simulink model "HeatExchanger_digital"  (Simulink 8.1)
settings: Solver=ode4  StartTime=0.0  StopTime=250  FixedStep=delta_t  RelTol=1e-3
values from neighbouring files (symbols this model uses):
  delta_t = 1 / sensor_sampling_rate    (= 0.1)    [HeatExchanger_ps.m]
  ki = 1.2    [HeatExchanger_ps.m]    (also in hxpumpcode.m = 1; hxpumpcodesanity.m; noErrornoDelay.mat = 1)
  kp = 4.995    [HeatExchanger_ps.m]    (also in hxpumpcode.m = 4; hxpumpcodesanity.m; noErrornoDelay.mat = 4)
  Sv_mh = 0.05    [HeatExchanger_ps.m]    (also in hxpumpcode.m = params.Sv_mh; hxpumpcodesanity.m; noErrornoDelay.mat)
  Sv_thi = 5e-2    (= 0.05)    [HeatExchanger_ps.m]    (also in hxpumpcode.m = params.Sv_thi; hxpumpcodesanity.m; noErrornoDelay.mat)
  Sv_tho = 0.1    [HeatExchanger_ps.m]    (also in hxpumpcode.m = params.Sv_tho; hxpumpcodesanity.m; noErrornoDelay.mat)
  Ts = delta_t    (= 0.1)    [HeatExchanger_ps.m]    (also in hxpumpcode.m = params.Ts; hxpumpcodesanity.m; noErrornoDelay.mat)
libraries: simulink x4, powerlib_meascontrol x3
settings Model: Creator=Rhine  LastModifiedBy=LabUser
settings DataIOCC: LimitDataPoints=off
settings GRTTargetCC: CodeReplacementLibrary=None  CPPClassGenCompliant=on

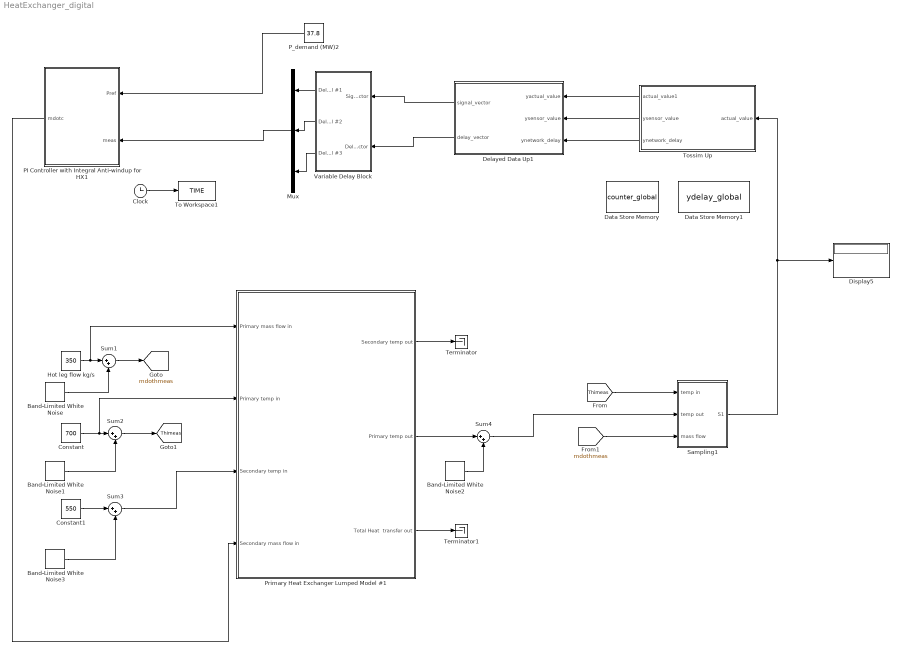
== system HeatExchanger_digital ==
  Band-Limited White Noise : simulink/Sources/Band-Limited White Noise  Cov=Sv_thi*Ts  Ts=Ts  seed=[34567]
  Band-Limited White Noise1 : simulink/Sources/Band-Limited White Noise  Cov=Sv_mh*Ts  Ts=Ts  seed=[11111]
  Band-Limited White Noise2 : simulink/Sources/Band-Limited White Noise  Cov=Sv_tho*Ts  Ts=Ts  seed=[45678]
  Band-Limited White Noise3 : simulink/Sources/Band-Limited White Noise  Cov=0  Ts=Ts  seed=[23341]
  Clock : Clock
  Constant : Constant  Value=700
  Constant1 : Constant  Value=550
  Data Store Memory : DataStoreMemory  DataStoreName=counter_global  ReadBeforeWriteMsg=warning  WriteAfterWriteMsg=warning  WriteAfterReadMsg=warning  OutDataTypeStr=int32
  Data Store Memory1 : DataStoreMemory  DataStoreName=ydelay_global  ReadBeforeWriteMsg=warning  WriteAfterWriteMsg=warning  WriteAfterReadMsg=warning  InitialValue=ones(10,1)  OutDataTypeStr=int32
  Delayed Data Up1 : MATLAB Function  TreatAsAtomicUnit=on  SystemSampleTime=0.1
  Display5 : Display
  Hot leg flow kg/s : Constant  Value=350
  Mux : Mux  Inputs=3
  PI Controller with Integral Anti-windup for HX1 : Subsystem
  P_demand (MW)2 : Constant  Value=37.8
  Primary Heat Exchanger Lumped Model #1 : Subsystem
  Sampling1 : Subsystem
  Sum{1..4} (4 alike) : Sum  Inputs=|++
  Terminator : Terminator
  Terminator1 : Terminator
  To Workspace1 : ToWorkspace  VariableName=TIME  SampleTime=-1
  Tossim Up : MATLAB Function  TreatAsAtomicUnit=on  SystemSampleTime=0.1
  Variable Delay Block : Subsystem
  tag scope: Thimeas=global, mdothmeas=global
  wires:
  Clock/1 -> To Workspace1/1
  Tossim Up/1(actual_value1) -> Delayed Data Up1/1(yactual_value)
  Sampling1/1(S1) -> Tossim Up/1(actual_value), Display5/1
  PI Controller with Integral Anti-windup for HX1/1(mdotc) -> Primary Heat Exchanger Lumped Model #1/4(Secondary mass flow in)
  Delayed Data Up1/1(signal_vector) -> Variable Delay Block/1(Signal vector)
  Tossim Up/2(ysensor_value) -> Delayed Data Up1/2(ysensor_value)
  Tossim Up/3(ynetwork_delay) -> Delayed Data Up1/3(ynetwork_delay)
  Delayed Data Up1/2(delay_vector) -> Variable Delay Block/2(Delay vector)
  P_demand (MW)2/1 -> PI Controller with Integral Anti-windup for HX1/1(Pref)
  Hot leg flow kg/s/1 -> Primary Heat Exchanger Lumped Model #1/1(Primary mass flow in), Sum1/1
  Constant/1 -> Primary Heat Exchanger Lumped Model #1/2(Primary temp in), Sum2/1
  Constant1/1 -> Sum3/1
  Sum3/1 -> Primary Heat Exchanger Lumped Model #1/3(Secondary temp in)
  Primary Heat Exchanger Lumped Model #1/1(Secondary temp out) -> Terminator/1
  Primary Heat Exchanger Lumped Model #1/3("Total Heat  transfer out ") -> Terminator1/1
  Sum1/1 -> [mdothmeas]
  Sum2/1 -> [Thimeas]
  [Thimeas] -> Sampling1/1(temp in)
  [mdothmeas] -> Sampling1/3(mass flow)
  Primary Heat Exchanger Lumped Model #1/2(Primary temp out) -> Sum4/1
  Band-Limited White Noise/1 -> Sum1/2
  Band-Limited White Noise1/1 -> Sum2/2
  Band-Limited White Noise2/1 -> Sum4/2
  Sum4/1 -> Sampling1/2(temp out)
  Band-Limited White Noise3/1 -> Sum3/2
  Variable Delay Block/1(Delayed signal #1) -> Mux/1
  Variable Delay Block/2(Delayed signal #2) -> Mux/2
  Variable Delay Block/3(Delayed signal #3) -> Mux/3
  Mux/1 -> PI Controller with Integral Anti-windup for HX1/2(meas)

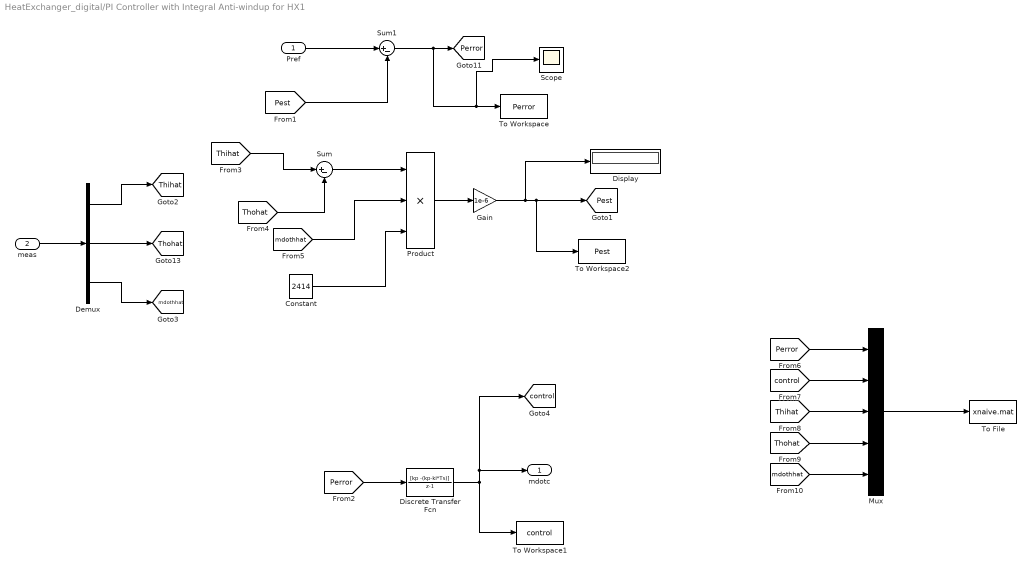
== system HeatExchanger_digital/PI Controller with Integral Anti-windup for HX1 ==
  Pref : Inport
  meas : Inport  Port=2
  Constant : Constant  Value=2414  SampleTime=Ts
  Demux : Demux  Outputs=3
  Discrete Transfer Fcn : DiscreteTransferFcn  Numerator=[kp -(kp-ki*Ts)]  Denominator=[1 -1]  InitialStates=20  SampleTime=Ts
  Display : Display
  Gain : Gain  Gain=1e-6
  Mux : Mux  Inputs=5
  Product : Product  Inputs=3
  Scope : Scope
  Sum : Sum  Inputs=|+-
  Sum1 : Sum  Inputs=|+-
  To File : ToFile  Filename=xnaive.mat  MatrixName=xnaive
  To Workspace : ToWorkspace  VariableName=Perror  SampleTime=-1
  To Workspace1 : ToWorkspace  VariableName=control  SampleTime=-1
  To Workspace2 : ToWorkspace  VariableName=Pest  SampleTime=-1
  mdotc : Outport
  tag scope: Perror=global, Pest=global, Thihat=global, Thohat=global, control=global, mdothhat=global
  wires:
  [Thohat] -> Sum/2
  [mdothhat] -> Product/2
  Sum/1 -> Product/1
  Constant/1 -> Product/3
  Product/1 -> Gain/1
  Pref/1 -> Sum1/1
  Gain/1 -> Display/1, To Workspace2/1, [Pest]
  [Pest] -> Sum1/2
  Sum1/1 -> To Workspace/1, Scope/1, [Perror]
  Discrete Transfer Fcn/1 -> [control], mdotc/1, To Workspace1/1
  [Perror] -> Discrete Transfer Fcn/1
  [Thihat] -> Sum/1
  Demux/3 -> [mdothhat]
  Demux/1 -> [Thihat]
  Demux/2 -> [Thohat]
  meas/1 -> Demux/1
  [Perror] -> Mux/1
  [control] -> Mux/2
  Mux/1 -> To File/1
  [mdothhat] -> Mux/5
  [Thohat] -> Mux/4
  [Thihat] -> Mux/3

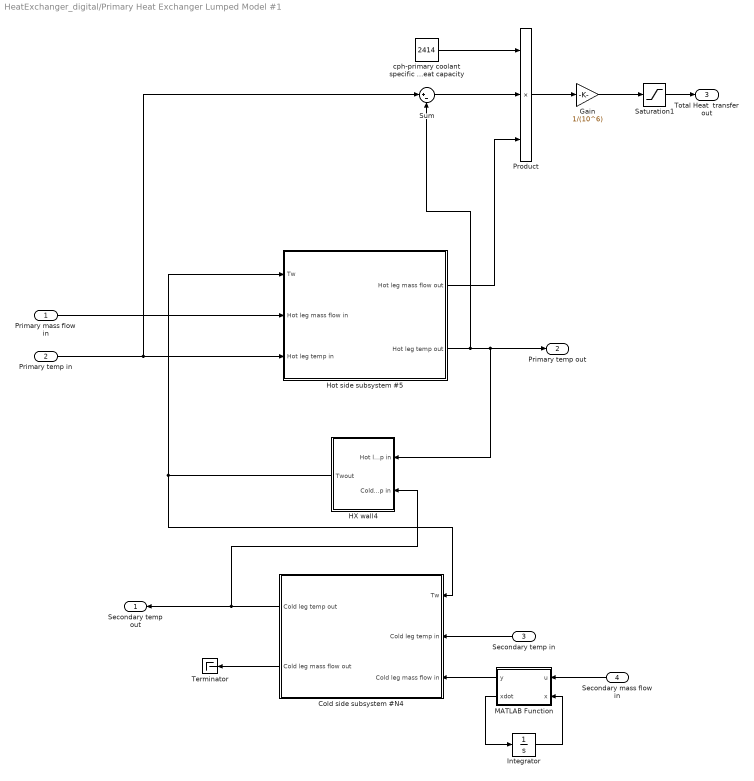
== system HeatExchanger_digital/Primary Heat Exchanger Lumped Model #1 ==
  Primary mass flow in : Inport
  Primary temp in : Inport  Port=2
  Secondary temp in : Inport  Port=3
  Secondary mass flow in : Inport  Port=4
  Cold side subsystem #N4 : Subsystem
  Gain : Gain  Gain=1/(10^6)
  HX wall4 : Subsystem
  Hot side subsystem #5 : Subsystem
  Integrator : Integrator  InitialCondition=250
  MATLAB Function : MATLAB Function  TreatAsAtomicUnit=on
  Product : Product  Inputs=3
  Saturation1 : Saturate  UpperLimit=inf  LowerLimit=0
  Sum : Sum  Inputs=|+-
  Terminator : Terminator
  cph-primary coolant specific heat capacity : Constant  Value=2414
  Secondary temp out : Outport
  Primary temp out : Outport  Port=2
  "Total Heat  transfer out " : Outport  Port=3
  wires:
  Cold side subsystem #N4/1(Cold leg temp out) -> Secondary temp out/1, HX wall4/2(Cold leg temp in)
  Cold side subsystem #N4/2(Cold leg mass flow out) -> Terminator/1
  Primary mass flow in/1 -> Hot side subsystem #5/2(Hot leg mass flow in)
  Primary temp in/1 -> Hot side subsystem #5/3(Hot leg temp in), Sum/1
  Secondary mass flow in/1 -> MATLAB Function/1(u)
  Secondary temp in/1 -> Cold side subsystem #N4/2(Cold leg temp in)
  HX wall4/1(Twout) -> Cold side subsystem #N4/1(Tw), Hot side subsystem #5/1(Tw)
  Hot side subsystem #5/1(Hot leg mass flow out) -> Product/3
  Hot side subsystem #5/2(Hot leg temp out) -> HX wall4/1(Hot leg temp in), Primary temp out/1, Sum/2
  cph-primary coolant specific heat capacity/1 -> Product/1
  Sum/1 -> Product/2
  Product/1 -> Gain/1
  Gain/1 -> Saturation1/1
  MATLAB Function/1(y) -> Cold side subsystem #N4/3(Cold leg mass flow in)
  Saturation1/1 -> "Total Heat  transfer out "/1
  MATLAB Function/2(xdot) -> Integrator/1
  Integrator/1 -> MATLAB Function/2(x)

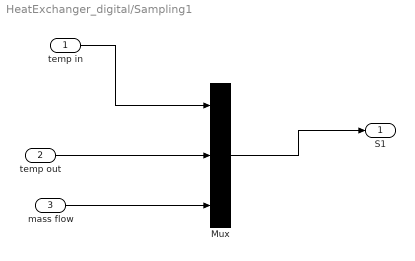
== system HeatExchanger_digital/Sampling1 ==
  temp in : Inport
  temp out : Inport  Port=2
  mass flow : Inport  Port=3
  Mux : Mux  Inputs=3
  S1 : Outport
  wires:
  temp in/1 -> Mux/1
  temp out/1 -> Mux/2
  mass flow/1 -> Mux/3
  Mux/1 -> S1/1

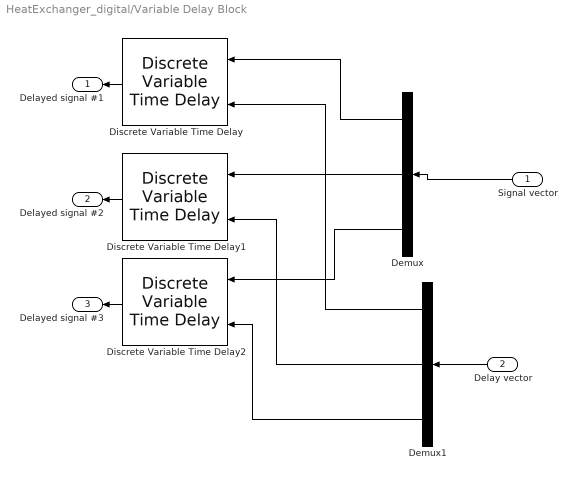
== system HeatExchanger_digital/Variable Delay Block ==
  Signal vector : Inport
  Delay vector : Inport  Port=2
  Demux : Demux  Outputs=3
  Demux1 : Demux  Outputs=3
  Discrete Variable Time Delay : powerlib_meascontrol/Additional Components/Discrete Variable Time Delay  MaxDelay=2  InitialValue=700  Ts=delta_t  DFT=on
  Discrete Variable Time Delay1 : powerlib_meascontrol/Additional Components/Discrete Variable Time Delay  MaxDelay=2  InitialValue=650.29  Ts=delta_t  DFT=on
  Discrete Variable Time Delay2 : powerlib_meascontrol/Additional Components/Discrete Variable Time Delay  MaxDelay=2  InitialValue=350  Ts=delta_t  DFT=on
  Delayed signal #1 : Outport
  Delayed signal #2 : Outport  Port=2
  Delayed signal #3 : Outport  Port=3
  wires:
  Discrete Variable Time Delay1/1 -> Delayed signal #2/1
  Demux1/3 -> Discrete Variable Time Delay2/2
  Demux1/2 -> Discrete Variable Time Delay1/2
  Discrete Variable Time Delay2/1 -> Delayed signal #3/1
  Demux/3 -> Discrete Variable Time Delay2/1
  Demux/1 -> Discrete Variable Time Delay/1
  Demux1/1 -> Discrete Variable Time Delay/2
  Discrete Variable Time Delay/1 -> Delayed signal #1/1
  Signal vector/1 -> Demux/1
  Demux/2 -> Discrete Variable Time Delay1/1
  Delay vector/1 -> Demux1/1

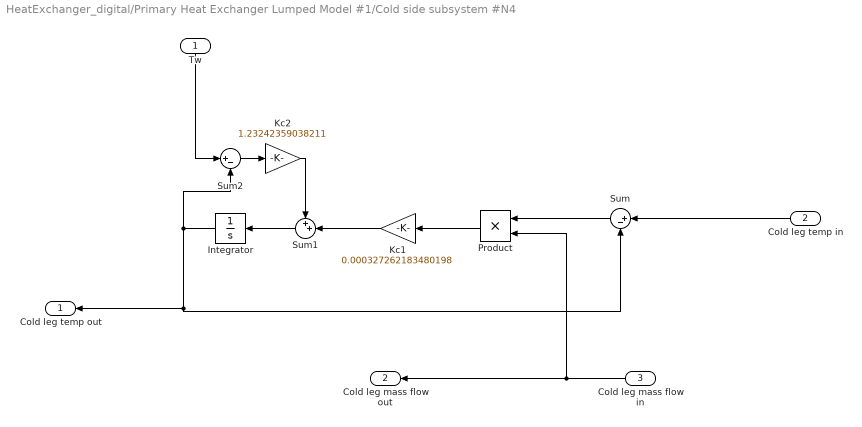
== system HeatExchanger_digital/Primary Heat Exchanger Lumped Model #1/Cold side subsystem #N4 ==
  Tw : Inport
  Cold leg temp in : Inport  Port=2
  Cold leg mass flow in : Inport  Port=3
  Integrator : Integrator  InitialCondition=638.4
  Kc1 : Gain  Gain=0.000327262183480198
  Kc2 : Gain  Gain=1.23242359038211
  Product : Product
  Sum : Sum  Inputs=|+-
  Sum1 : Sum  Inputs=++|
  Sum2 : Sum  Inputs=|+-
  Cold leg temp out : Outport
  Cold leg mass flow out : Outport  Port=2
  wires:
  Cold leg temp in/1 -> Sum/1
  Integrator/1 -> Sum/2, Cold leg temp out/1, Sum2/2
  Sum2/1 -> Kc2/1
  Sum/1 -> Product/1
  Kc2/1 -> Sum1/1
  Sum1/1 -> Integrator/1
  Cold leg mass flow in/1 -> Cold leg mass flow out/1, Product/2
  Product/1 -> Kc1/1
  Kc1/1 -> Sum1/2
  Tw/1 -> Sum2/1

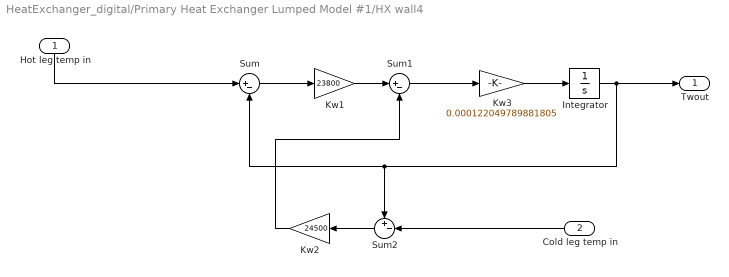
== system HeatExchanger_digital/Primary Heat Exchanger Lumped Model #1/HX wall4 ==
  Hot leg temp in : Inport
  Cold leg temp in : Inport  Port=2
  Integrator : Integrator  InitialCondition=644.3
  Kw1 : Gain  Gain=23800
  Kw2 : Gain  Gain=24500
  Kw3 : Gain  Gain=0.000122049789881805
  Sum : Sum  Inputs=|+-
  Sum1 : Sum  Inputs=|+-
  Sum2 : Sum  Inputs=+-|
  Twout : Outport
  wires:
  Sum2/1 -> Kw2/1
  Hot leg temp in/1 -> Sum/1
  Sum1/1 -> Kw3/1
  Cold leg temp in/1 -> Sum2/2
  Sum/1 -> Kw1/1
  Kw1/1 -> Sum1/1
  Kw3/1 -> Integrator/1
  Integrator/1 -> Twout/1, Sum2/1, Sum/2
  Kw2/1 -> Sum1/2

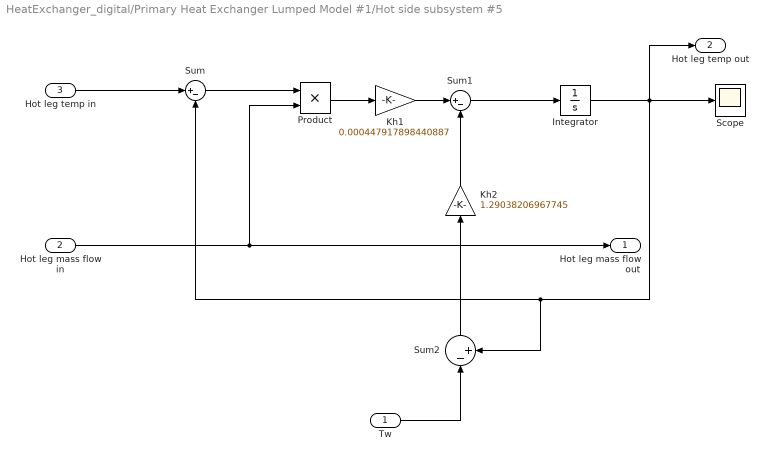
== system HeatExchanger_digital/Primary Heat Exchanger Lumped Model #1/Hot side subsystem #5 ==
  Tw : Inport
  Hot leg mass flow in : Inport  Port=2
  Hot leg temp in : Inport  Port=3
  Integrator : Integrator  InitialCondition=650.29
  Kh1 : Gain  Gain=0.000447917898440887
  Kh2 : Gain  Gain=1.29038206967745
  Product : Product
  Scope : Scope
  Sum : Sum  Inputs=|+-
  Sum1 : Sum  Inputs=|+-
  Sum2 : Sum  Inputs=|-+
  Hot leg mass flow out : Outport
  Hot leg temp out : Outport  Port=2
  wires:
  Product/1 -> Kh1/1
  Kh1/1 -> Sum1/1
  Sum1/1 -> Integrator/1
  Sum2/1 -> Kh2/1
  Kh2/1 -> Sum1/2
  Tw/1 -> Sum2/1
  Hot leg temp in/1 -> Sum/1
  Hot leg mass flow in/1 -> Hot leg mass flow out/1, Product/2
  Sum/1 -> Product/1
  Integrator/1 -> Hot leg temp out/1, Scope/1, Sum2/2, Sum/2

== matlab function Tossim Up ==
  data: actual_value1 output double; actual_value input double; ysensor_value output double; ydelay_global data_store_memory double; counter_global data_store_memory double; ynetwork_delay output double
function [actual_value1, ysensor_value, ynetwork_delay]  = Tossim_block(actual_value)

% Inputs:
% ymea: measurement from structure

% Outputs:
% ymea1: measurement output
% ydelay: delay traces

persistent sensor_value % delay trace
persistent i  
persistent network_array
% count
global ydelay_global
global counter_global

iterations = 3001;

% allow these matlab functions to be used in Embedded Matlab block
eml.extrinsic('python');
eml.extrinsic('num2str');
eml.extrinsic('str2num');
eml.extrinsic('delay_summary');
eml.extrinsic('disp');
%eml.extrinsic('ps_aggregation');
eml.extrinsic('ps_text');
eml.extrinsic('for');
eml.extrinsic('end');
eml.extrinsic('fgets');
eml.extrinsic('fopen');

if isempty(i)
    i = 0;
    
    % read "network_error_delay.txt" file
    network_array= zeros(iterations, 6);
    %file_fp = fopen('/Users/wangwenchen/wcps_apps/stepF_HX/simu.cfg');
    %filename = fgets(file_fp);
    %disp(filename);
    %fclose(file_fp);
    
    
    filename='noErrornoDelay.txt';
    
    
    %filename='/Users/wangwenchen/github/paper2_result/fault_model_1/schemeMICD_lpSample20_topoSample20/1_control_input.txt';
    text=fopen(filename);
    result=fgets(text);

    %network_array(1, :) = str2num(result);
    line_num=1;
    while ischar(result)
        if( line_num <=iterations)
            network_array(line_num, :) = str2num(result);
            result = fgets(text);
        else
            break;
        end

        line_num = line_num+1;

    end
    fclose(text);
    %disp(network_array);
end

%sen_num=structure.sen_num;

ysensor_value = [0 0 0]'; 
ynetwork_delay = [0 0 0]';



%call_count = 56; % number of slots + 1 (i.e., number of client calls made + 1) per TDMA schedule, +1 to have full 53 slots after %

%[resultz] = ps_aggregation(call_count);
i = i + 1;
%[resultz] = ps_text(i);
resultz=network_array(i, :);

%end_to_end_delivery_result_aggregated = sum(resultz);
%end_to_end_delivery_result_aggregated=resultz;

[sensor_value_tmp] = value_summary(resultz);
if i==1
    sensor_value_tmp=[1 1 1];
end
ysensor_value = sensor_value_tmp';

[network_delay_tmp] = network_delay_summary(resultz);
%disp(network_delay)
ynetwork_delay=network_delay_tmp';

disp('sensor_value')
disp(ysensor_value')
%disp('network delay')
%disp(ynetwork_delay')
disp('------------i------------')
disp(i)

%last_emergency_instance = ymea';
sensor_value = ysensor_value;


actual_value1 = [0 0 0]'; %3 sensors
actual_value1 = actual_value;


for h_yg = 1:3
    ydelay_global(h_yg, 1) = ysensor_value(h_yg, 1);
end

disp('Plant 1, TOSSIM Uplink Block, is called');
counter_global = counter_global + 1;

== matlab function Primary Heat Exchanger Lumped Model #1/MATLAB Function ==
  data: u input double; y output double; x input double; xdot output double
function [y,xdot] = pump(u,x)
%#codegen

if u<0
    u=0;
else
end

xdot = -0.1*x + 0.1*u;

y = x;

== matlab function Delayed Data Up1 ==
  data: yactual_value input double; ysensor_value input double; ynetwork_delay input double; signal_vector output double; structure parameter double; delay_vector output double
function [signal_vector, delay_vector] = delay_block(yactual_value,ysensor_value, ynetwork_delay, structure)

% Inputs: 
% yactual_value: measurements output
% yactual_value: sensor value traces
% ynetwork_delay: delay traces
% structure: other necessary information 

% Outputs:
% signal_vector: sensor measurments
% delay_vector: delay value
persistent  i yin_d delay_v
persistent yin sensor_value num ynd_tmp
persistent last_senReading last_senDelay
%global yin_all ynd_all

eml.extrinsic('disp');
eml.extrinsic('putvar');



% sennum=5;  %number of the sensors
%step_count = 1000; %step_count
%sen_num=9;
% initialize parameters
if isempty(yin)
    i = structure.i;
    yin = structure.yin;    
    ynd_tmp= structure.ynd_tmp;

    yin_d = structure.yin_d; 
    delay_v = structure.delay_v;
    
    last_senReading = zeros(1,9);
    last_senDelay = zeros(1,9);
    
    %yin_all = structure.yin_all; %zeros (step count, sensor number)
    %ynd_all=structure.ynd_all;
    
    %yin_all = zeros(step_count+1,9); %zeros (step count, sensor number)
    %ynd_all=zeros(step_count+1,9);
    
    sensor_value = zeros(1,3);         %initialized
    sensor_value = ysensor_value';
    num = 0;
end

%yin_all = zeros(step_count+1,9); %zeros (step count, sensor number)
%ynd_all=zeros(step_count+1,9);

sensor_reading=[0 0 0];
sensor_delay=[0 0 0];
num = num+1;   

%get delay information 
% delay=zeros(1,10+1); 
sensor_value=ysensor_value';
    

%get value from "yactual_value" input
if num == 1
    for kk = 1:3
        last_senReading(kk) = yactual_value(kk); %offset=5
        last_senDelay(kk) = ynetwork_delay(kk);
    end 
end
%generate output value according to delay    
for j=1:3
    if sensor_value(1,j)~=88
        last_senReading(j) = yactual_value(j);
        last_senDelay(j) = ynetwork_delay(j);
        yin(j) = last_senReading(j);  %packet receive
        ynd_tmp(j)=last_senDelay(j);
        
    else
        if num>1 
             yin(j)=last_senReading(j); %if lost, set it to previous value
             last_senReading(j)=last_senReading(j);
             ynd_tmp(j)=last_senDelay(j)+0.1;
             last_senDelay(j)=last_senDelay(j)+0.1;
        end        
    end
end

avg_delay=0.0;

for kk = 1:3
    %sensor_reading(kk)= yin_all(num,kk); %offset=5
    %sensor_delay(kk) = ynd_all(num,kk);
    avg_delay =last_senDelay(kk)+avg_delay;

end

avg_delay = avg_delay/3.0;
fileID = fopen('sensor_data.txt','a');
fprintf(fileID, '%f\n', avg_delay);
fclose(fileID);

%putvar(yin_all, ynd_all);

%structure.yin_all=yin_all;
%structure.ynd_all=ynd_all;

yin_d = yin';
delay_v = ynd_tmp';
%delay_v = ynd_tmp'/3;
%delay_v = [0,0,0]';

signal_vector = yin_d;

delay_vector = delay_v;

disp('actual value')
disp(yactual_value);

disp('converted sensor_value')
disp(signal_vector')
disp('converted network delay')
disp(delay_vector')
disp('---------------num-------------')
disp(num)

% disp('plant2');

% yout_delay'
i = i+1;
